simulink model "ModelloNonLineare"  (R2023a)
settings: Solver=VariableStepAuto  StartTime=0.0  StopTime=100  RelTol=1e-3
values from neighbouring files (symbols this model uses):
  Ad = 60    [Script_Dirigibile.m]
  b = 20    [Script_Dirigibile.m]
  c = 12.5    [Script_Dirigibile.m]
  Cd = 0.05    [Script_Dirigibile.m]
  g = 9.81    [Script_Dirigibile.m]
  k = 15    [Script_Dirigibile.m]
  m = 1000    [Script_Dirigibile.m]
  rho_a = 1.225    [Script_Dirigibile.m]
  T_a = 288.15    [Script_Dirigibile.m]
  V = 4000    [Script_Dirigibile.m]
  x0 = [0 0 T_a]'    [Script_Dirigibile.m]
settings Model: Creator=giuco  LastModifiedBy=giuco

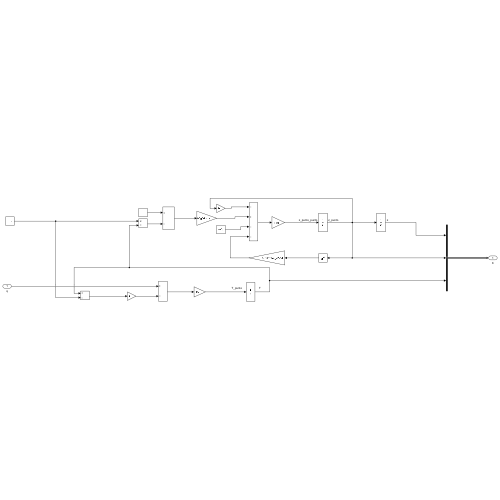
[thumbnail: Simulink's stored preview of the top-level diagram]
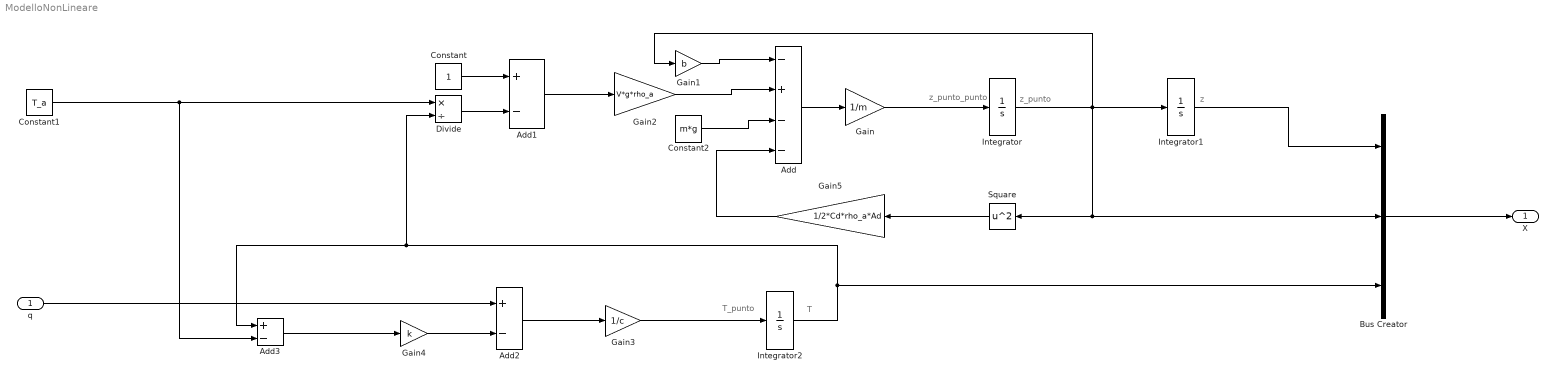
== system ModelloNonLineare ==
  note: T
  note: T_punto
  note: z
  note: z_punto
  note: z_punto_punto
  q : Inport
  Add : Sum  Inputs=-+--
  Add1 : Sum  Inputs=+-
  Add2 : Sum  Inputs=+-
  Add3 : Sum  Inputs=+-
  Bus Creator : BusCreator  Inputs=3
  Constant : Constant
  Constant1 : Constant  Value=T_a
  Constant2 : Constant  Value=m*g
  Divide : Product  Inputs=*/
  Gain : Gain  Gain=1/m
  Gain1 : Gain  Gain=b
  Gain2 : Gain  Gain=V*g*rho_a
  Gain3 : Gain  Gain=1/c
  Gain4 : Gain  Gain=k
  Gain5 : Gain  Gain=1/2*Cd*rho_a*Ad
  Integrator : Integrator  InitialCondition=x0(2)
  Integrator1 : Integrator  InitialCondition=x0(1)
  Integrator2 : Integrator  InitialCondition=x0(3)
  Square : Math  Operator=square
  X : Outport
  wires:
  Integrator/1 -> Square/1, Bus Creator/2, Gain1/1, Integrator1/1
  Gain/1 -> Integrator/1
  Add/1 -> Gain/1
  Gain1/1 -> Add/1
  Gain3/1 -> Integrator2/1
  Integrator2/1 -> Bus Creator/3, Add3/1, Divide/2
  Constant/1 -> Add1/1
  Divide/1 -> Add1/2
  Constant1/1 -> Add3/2, Divide/1
  Gain2/1 -> Add/2
  Constant2/1 -> Add/3
  Add2/1 -> Gain3/1
  q/1 -> Add2/1
  Gain4/1 -> Add2/2
  Add3/1 -> Gain4/1
  Bus Creator/1 -> X/1
  Add1/1 -> Gain2/1
  Square/1 -> Gain5/1
  Gain5/1 -> Add/4
  Integrator1/1 -> Bus Creator/1
